simulink model "DC_Motor"  (R2025a)
settings: Solver=ode4  StartTime=0.0  StopTime=12  FixedStep=0.001  RelTol=1e-3
values from neighbouring files (symbols this model uses):
  A = [-R/L -Ke/L ; Kt/J 0]    [MotoreDC.m]    (also in MotoreDC_pt2.m = -beta./J)
  B = [1/L 0 ; 0 -1/J]    [MotoreDC.m]    (also in MotoreDC_pt2.m = 625000)
  C = eye(2)    [MotoreDC.m]    (also in MotoreDC_pt2.m = 1)
  C_den_I = C_tfDen(1,:)    [MotoreDC.m]
  C_den_W = C_tfDen(1,:)    [MotoreDC.m]
  C_num_I = C_tfNum(1,:)    [MotoreDC.m]
  C_num_W = C_tfNum(2,:)    [MotoreDC.m]
  Cr = [Cr_Stall; Cr_Rated ; Cr_noLoad]    [MotoreDC.m]
  Cr_noLoad = 0.0    (= 0)    [MotoreDC.m]
  Cr_pt4 = (0:1:6)/100    [MotoreDC.m]
  Cr_Rated = 2.0e-2    (= 0.02)    [MotoreDC.m]
  Cr_Stall = 6.6e-2    (= 0.066)    [MotoreDC.m]
  D = zeros(2)    [MotoreDC.m]    (also in MotoreDC_pt2.m = 0)
  J = 16e-7    (= 1.6e-06)    [MotoreDC.m]    (also in MotoreDC_pt2.m)
  Ke = 0.025    [MotoreDC.m]    (also in MotoreDC_pt2.m)
  Kt = 2.5e-2    (= 0.025)    [MotoreDC.m]    (also in MotoreDC_pt2.m)
  L = 6.2e-3    (= 0.0062)    [MotoreDC.m]    (also in MotoreDC_pt2.m)
  R = 4.4    [MotoreDC.m]    (also in MotoreDC_pt2.m)
  V_den_I = V_tfDen(1,:)    [MotoreDC.m]
  V_den_W = V_tfDen(1,:)    [MotoreDC.m]
  V_num_I = V_tfNum(1,:)    [MotoreDC.m]
  V_num_W = V_tfNum(2,:)    [MotoreDC.m]
  V_pt4 = 0:2:12    [MotoreDC.m]
libraries: simulink x3
settings Model: Creator=Mattia  LastModifiedBy=Mattia

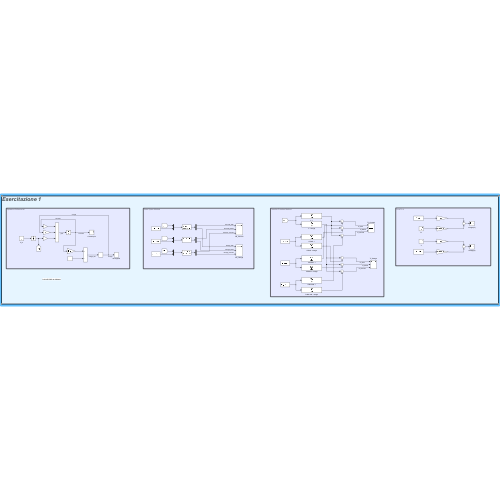
[thumbnail: Simulink's stored preview of the top-level diagram]
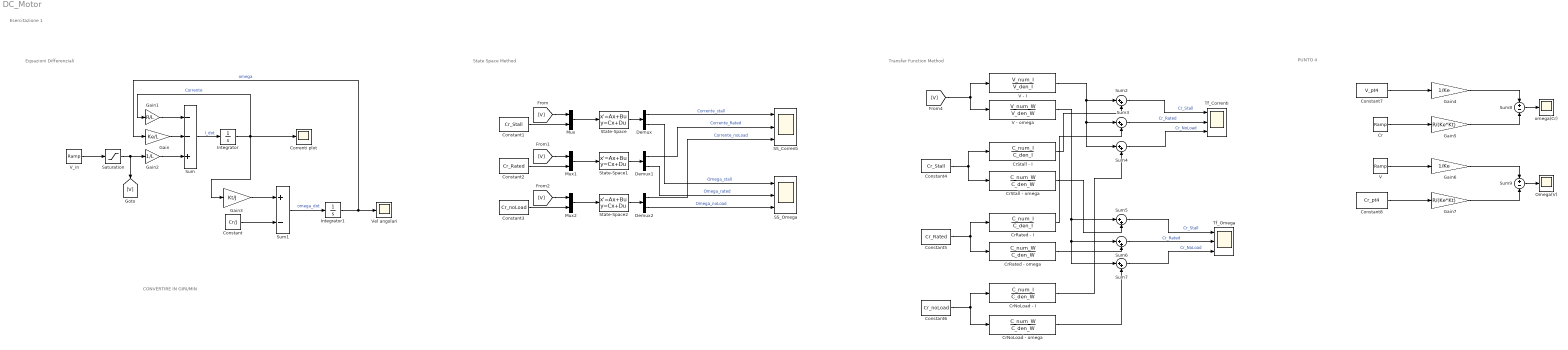
== system DC_Motor ==
  note: CONVERTIRE IN GIRI/MIN
  note: Esercitazione 1
  note: PUNTO 4
  note: State Space Method
  note: Equazioni Differenziali
  note: Transfer Function Method
  Constant : Constant  Value=Cr/J
  Constant1 : Constant  Value=Cr_Stall
  Constant2 : Constant  Value=Cr_Rated
  Constant3 : Constant  Value=Cr_noLoad
  Constant4 : Constant  Value=Cr_Stall
  Constant5 : Constant  Value=Cr_Rated
  Constant6 : Constant  Value=Cr_noLoad
  Constant7 : Constant  Value=V_pt4
  Constant8 : Constant  Value=Cr_pt4
  Correnti plot : Scope
      settings: ActiveDisplayYMinimum=-0.59781458586792979  ActiveDisplayYMaximum=4.6699910044862092
  Cr : simulink/Sources/Ramp  slope=1  start=0  InitialOutput=0
  CrNoLoad - I : TransferFcn  Numerator=C_num_I  Denominator=C_den_W
  CrNoLoad - omega : TransferFcn  Numerator=C_num_W  Denominator=C_den_W
  CrRated - I : TransferFcn  Numerator=C_num_I  Denominator=C_den_I
  CrRated - omega : TransferFcn  Numerator=C_num_W  Denominator=C_den_W
  CrStall - I : TransferFcn  Numerator=C_num_I  Denominator=C_den_I
  CrStall - omega : TransferFcn  Numerator=C_num_W  Denominator=C_den_W
  Demux : Demux  Outputs=2
  Demux1 : Demux  Outputs=2
  Demux2 : Demux  Outputs=2
  Gain : Gain  Gain=Ke/L
  Gain1 : Gain  Gain=R/L
  Gain2 : Gain  Gain=1/L
  Gain3 : Gain  Gain=Kt/J
  Gain4 : Gain  Gain=1/Ke
  Gain5 : Gain  Gain=R/(Ke*Kt)
  Gain6 : Gain  Gain=1/Ke
  Gain7 : Gain  Gain=R/(Ke*Kt)
  Integrator : Integrator
  Integrator1 : Integrator
  Mux : Mux  Inputs=2
  Mux1 : Mux  Inputs=2
  Mux2 : Mux  Inputs=2
  Omega(V) : Scope
      settings: ActiveDisplayYMinimum=-1558.5606535253671  ActiveDisplayYMaximum=1279.0044206845635  DataLoggingVariableName=ScopeData7
  SS_Correnti : Scope  NumInputPorts=3
      settings: ActiveDisplayYMinimum=-0.995510177466328  ActiveDisplayYMaximum=3.1793403949224803  DataLoggingVariableName=ScopeData2
  SS_Omega : Scope  NumInputPorts=3
      settings: ActiveDisplayYMinimum=-532.08847046569747  ActiveDisplayYMaximum=637.24182059732289  DataLoggingVariableName=ScopeData3
  Saturation : Saturate  UpperLimit=12  LowerLimit=0
  State-Space : StateSpace  A=A  B=B  C=C  D=D  InitialCondition=0
  State-Space1 : StateSpace  A=A  B=B  C=C  D=D  InitialCondition=0
  State-Space2 : StateSpace  A=A  B=B  C=C  D=D  InitialCondition=0
  Sum : Sum  Inputs=--+
  Sum1 : Sum  Inputs=+-
  Sum{2..7} (6 alike) : Sum  Inputs=|++
  Sum8 : Sum  Inputs=+-
  Sum9 : Sum  Inputs=+-
  Tf_Correnti : Scope  NumInputPorts=3
      settings: ActiveDisplayYMinimum=-2.7184675270542407  ActiveDisplayYMaximum=1.7071401269619766  DataLoggingVariableName=ScopeData5
  Tf_Omega : Scope  NumInputPorts=3
      settings: ActiveDisplayYMinimum=-452.4737682571506  ActiveDisplayYMaximum=404.30195887525048  DataLoggingVariableName=ScopeData6
  V : simulink/Sources/Ramp  slope=1  start=0  InitialOutput=0
  V - I : TransferFcn  Numerator=V_num_I  Denominator=V_den_I
  V - omega : TransferFcn  Numerator=V_num_W  Denominator=V_den_W
  V_in : simulink/Sources/Ramp  slope=1  start=0  InitialOutput=0
  Vel angolari : Scope
      settings: ActiveDisplayYMinimum=-860.15716514113865  ActiveDisplayYMaximum=1103.0167950152154
  omega(Cr) : Scope
      settings: ActiveDisplayYMinimum=-1558.5606535253671  ActiveDisplayYMaximum=1279.0044206845635  DataLoggingVariableName=ScopeData4
  wires:
  Gain/1 -> Sum/2
  Gain2/1 -> Sum/3
  Gain1/1 -> Sum/1
  Sum/1 -> Integrator/1  "I_dot"
  Integrator/1 -> Gain3/1, Gain1/1, Correnti plot/1  "Corrente"
  Gain3/1 -> Sum1/1
  Constant/1 -> Sum1/2
  Sum1/1 -> Integrator1/1  "omega_dot"
  Integrator1/1 -> Gain/1, Vel angolari/1  "omega"
  V_in/1 -> Saturation/1
  Saturation/1 -> Gain2/1, [V]
  [V] -> Mux/1
  Mux/1 -> State-Space/1
  Constant1/1 -> Mux/2
  State-Space/1 -> Demux/1
  Demux/1 -> SS_Correnti/1  "Corrente_stall"
  Demux/2 -> SS_Omega/1  "Omega_stall"
  [V] -> Mux1/1
  Demux1/1 -> SS_Correnti/2  "Corrente_Rated"
  Constant2/1 -> Mux1/2
  Mux1/1 -> State-Space1/1
  Demux1/2 -> SS_Omega/2  "Omega_rated"
  State-Space1/1 -> Demux1/1
  [V] -> Mux2/1
  Demux2/1 -> SS_Correnti/3  "Corrente_noLoad"
  Constant3/1 -> Mux2/2
  Mux2/1 -> State-Space2/1
  Demux2/2 -> SS_Omega/3  "Omega_noLoad"
  State-Space2/1 -> Demux2/1
  [V] -> V - I/1, V - omega/1
  Constant5/1 -> CrRated - I/1, CrRated - omega/1
  Constant6/1 -> CrNoLoad - I/1, CrNoLoad - omega/1
  Constant4/1 -> CrStall - I/1, CrStall - omega/1
  V - I/1 -> Sum3/1, Sum4/1, Sum2/1
  V - omega/1 -> Sum7/1, Sum6/1, Sum5/1
  CrStall - I/1 -> Sum2/2
  CrRated - I/1 -> Sum3/2
  CrNoLoad - I/1 -> Sum4/2
  CrStall - omega/1 -> Sum5/2
  CrRated - omega/1 -> Sum6/2
  CrNoLoad - omega/1 -> Sum7/2
  Sum2/1 -> Tf_Correnti/1  "Cr_Stall"
  Sum3/1 -> Tf_Correnti/2  "Cr_Rated"
  Sum4/1 -> Tf_Correnti/3  "Cr_NoLoad"
  Sum5/1 -> Tf_Omega/1  "Cr_Stall"
  Sum6/1 -> Tf_Omega/2  "Cr_Rated"
  Sum7/1 -> Tf_Omega/3  "Cr_NoLoad"
  Constant7/1 -> Gain4/1
  Gain4/1 -> Sum8/1
  Gain5/1 -> Sum8/2
  Sum8/1 -> omega(Cr)/1
  Cr/1 -> Gain5/1
  V/1 -> Gain6/1
  Sum9/1 -> Omega(V)/1
  Gain6/1 -> Sum9/1
  Gain7/1 -> Sum9/2
  Constant8/1 -> Gain7/1
